simulink model "Rotor_Position_Hall_AD"  (R2020a)
settings: Solver=FixedStepAuto  StartTime=0.0  StopTime=10.0  FixedStep=Ts_Sensor  RelTol=1e-3
undefined symbols (not defined in the file): ADCBit, Hall_Gain, Hall_Offset, Ts_Sensor, Vcc
settings Model: Creator=BEDNASA  LastModifiedBy=BEDNASA

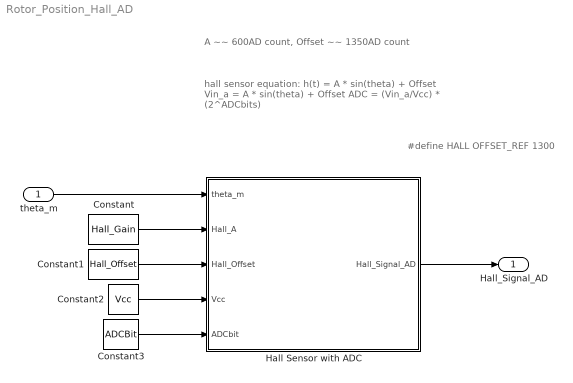
== system Rotor_Position_Hall_AD ==
  note: #define HALL OFFSET_REF 1300
  note: A ~~ 600AD count, Offset ~~ 1350AD count
  note: hall sensor equation: h(t) = A * sin(theta) + Offset
      |
      | Vin_a = A * sin(theta) + Offset
      |
      | ADC = (Vin_a/Vcc) * (2^ADCbits)
  theta_m : Inport
  Constant : Constant  Value=Hall_Gain
  Constant1 : Constant  Value=Hall_Offset
  Constant2 : Constant  Value=Vcc
  Constant3 : Constant  Value=ADCBit
  Hall Sensor with ADC : MATLAB Function  TreatAsAtomicUnit=on  SystemSampleTime=Ts_Sensor
  Hall_Signal_AD : Outport
  wires:
  theta_m/1 -> Hall Sensor with ADC/1(theta_m)
  Hall Sensor with ADC/1(Hall_Signal_AD) -> Hall_Signal_AD/1
  Constant/1 -> Hall Sensor with ADC/2(Hall_A)
  Constant1/1 -> Hall Sensor with ADC/3(Hall_Offset)
  Constant2/1 -> Hall Sensor with ADC/4(Vcc)
  Constant3/1 -> Hall Sensor with ADC/5(ADCbit)

== matlab function Rotor_Position_Hall_AD/Hall Sensor with ADC ==
  data: theta_m input; Hall_Signal_AD output; Hall_A input; Hall_Offset input; Vcc input; ADCbit input
function Hall_Signal_AD = fcn(theta_m, Hall_A, Hall_Offset, Vcc, ADCbit)
%% Hall sensor model with ADC
% Hall sensor equation h = A * sin(theta_m) + Offset
% h - output signal in [V]
% Vcc - ADC reference voltage
% ADCbit - ADC bits

V_out_hall = Hall_A * sin(theta_m) + Hall_Offset;

if (V_out_hall > Vcc)
    V_out_hall = Vcc;
elseif (V_out_hall < 0)
    V_out_hall = 0;
end

%% AD Counts
Hall_Signal_AD = round((V_out_hall/Vcc) * (2^ADCbit));
